simulink model "schema_elec_causal"  (R2016b)
settings: Solver=VariableStepAuto  StartTime=0.0  StopTime=10.0  RelTol=1e-3
values from neighbouring files (symbols this model uses):
  C = 9.038    [declaration_des_variables.m]
undefined symbols (not defined in the file or in its folder): L, R
settings Model: Creator=emiliendurif  LastModifiedBy=emiliendurif

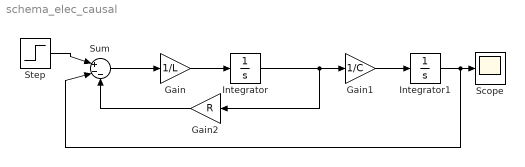
== system schema_elec_causal ==
  Gain : Gain  Gain=1/L
  Gain1 : Gain  Gain=1/C
  Gain2 : Gain  Gain=R
  Integrator : Integrator
  Integrator1 : Integrator
  Scope : Scope
  Step : Step  SampleTime=0
  Sum : Sum  Inputs=|+--
  wires:
  Integrator/1 -> Gain2/1, Gain1/1
  Gain1/1 -> Integrator1/1
  Gain/1 -> Integrator/1
  Sum/1 -> Gain/1
  Gain2/1 -> Sum/3
  Step/1 -> Sum/1
  Integrator1/1 -> Sum/2, Scope/1
